simulink library "inp"  (R2024a)
settings: Solver=VariableStepAuto  StartTime=0.0  StopTime=10.0  RelTol=1e-3
undefined symbols (not defined in the file): C_TASK_5MS_S, TRUE
libraries: FVT_lib x54, hcu_lib x1
(part 1 of 2)
settings Model: Creator=13168  LastModifiedBy=FVT22063
settings SolverCC: AlgebraicLoopSolver=TrustRegion
settings DataIOCC: SaveFormat=Array  SignalLoggingSaveFormat=ModelDataLogs  ReturnWorkspaceOutputs=off
settings OptimizationCC: BlockReduction=off  BooleanDataType=off
settings DebuggingCC: SaveWithParameterizedLinksMsg=none  UnderspecifiedInitializationDetection=Classic  MergeDetectMultiDrivingBlocksExec=none  SignalResolutionControl=TryResolveAllWithWarning  UnconnectedInputMsg=warning  UnconnectedOutputMsg=warning  UnconnectedLineMsg=warning
settings HardwareCC: TargetUnknown=on
settings ModelReferenceCC: EnableRefExpFcnMdlSchedulingChecks=on  PropagateSignalLabelsOutOfModel=off
settings SFSimCC: SimUseLocalCustomCode=off
settings RTWCC: GPUComputeCapability=3.5  DLArmComputeVersion=19.05
settings ConfigComp: CovMetricSettings=dw  CovSaveCumulativeToWorkspaceVar=on  CovSaveSingleToWorkspaceVar=on

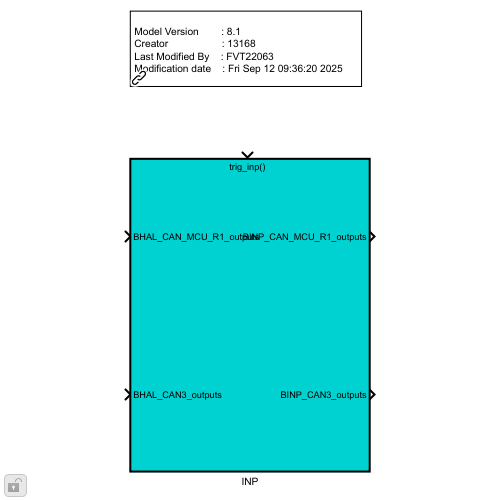
[thumbnail: Simulink's stored preview of the top-level diagram]
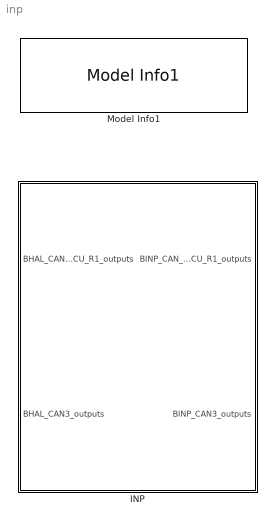
== system inp ==
  INP : Subsystem  TreatAsAtomicUnit=on
      settings: RTWSystemCode=Nonreusable function  RTWFcnNameOpts=Use subsystem name  RTWFileNameOpts=Use subsystem name
  Model Info1 : hcu_lib/Model Info1  BlockCM=None  Frame=on  DisplayStringWithTags=|  HorizontalTextAlignment=Left  LeftAlignmentValue=0.02  SourceBlockDiagram=hcu_lib  TagMaxNumber=20
      | Model Version        : %<ModelVersion>
      | Creator                   : %<Creator>
      | Last Modified By    : %<LastModifiedBy>
      | Modification date    : %<LastModificationDate>
      settings: SourceProductName=HCU Relative Block Library

== system inp/INP ==
  BHAL_CAN_MCU_R1_outputs : Inport  OutDataTypeStr=Bus: BHAL_CAN_MCU_R1_outputs
  BHAL_CAN3_outputs : Inport  Port=2  OutDataTypeStr=Bus: BHAL_CAN3_outputs
  CAN3 : Subsystem
  CAN_MCU_R1 : Subsystem
  BINP_CAN_MCU_R1_outputs : Outport  OutDataTypeStr=Bus: BINP_CAN_MCU_R1_outputs
  BINP_CAN3_outputs : Outport  Port=2  OutDataTypeStr=Bus: BINP_CAN3_outputs
  wires:
  BHAL_CAN_MCU_R1_outputs/1 -> CAN_MCU_R1/1(BHAL_CAN_MCU_R1_outputs)
  CAN_MCU_R1/1(INP_CAN_MCU_R1_outputs) -> BINP_CAN_MCU_R1_outputs/1
  BHAL_CAN3_outputs/1 -> CAN3/1(BHAL_CAN3_outputs)
  CAN3/1(INP_CAN3_outputs) -> BINP_CAN3_outputs/1

== system inp/INP/CAN3 ==
  BHAL_CAN3_outputs : Inport
  CommunicationCheck : Subsystem
  CreateBus : Subsystem
  SignalCheck : Subsystem
  ctasktime : Constant  Value=C_TASK_5MS_S  OutDataTypeStr=single
  INP_CAN3_outputs : Outport
  wires:
  CreateBus/1(BINP_outputs) -> INP_CAN3_outputs/1
  CommunicationCheck/1(inp_CanValid_bus) -> [inp_CanValid_bus], SignalCheck/1(inp_CanValid_bus)
  [inp_CanValid_bus] -> CreateBus/1(inp_CanValid_bus)
  BHAL_CAN3_outputs/1 -> CommunicationCheck/1(BHAL_outputs), SignalCheck/3(BHAL_outputs)
  SignalCheck/1(inp_Hal_bus) -> CreateBus/2(inp_Hal_bus)
  ctasktime/1 -> SignalCheck/2(TASK_TIME_S)

== system inp/INP/CAN_MCU_R1 ==
  BHAL_CAN_MCU_R1_outputs : Inport
  CommunicationCheck : Subsystem
  CreateBus : Subsystem
  SignalCheck : Subsystem
  ctasktime : Constant  Value=C_TASK_5MS_S  OutDataTypeStr=single
  INP_CAN_MCU_R1_outputs : Outport
  wires:
  CreateBus/1(BINP_outputs) -> INP_CAN_MCU_R1_outputs/1
  CommunicationCheck/1(inp_CanValid_bus) -> [inp_CanValid_bus], SignalCheck/1(inp_CanValid_bus)
  [inp_CanValid_bus] -> CreateBus/1(inp_CanValid_bus)
  BHAL_CAN_MCU_R1_outputs/1 -> CommunicationCheck/1(BHAL_outputs), SignalCheck/3(BHAL_outputs)
  SignalCheck/1(inp_Hal_bus) -> CreateBus/2(inp_Hal_bus)
  ctasktime/1 -> SignalCheck/2(TASK_TIME_S)

== system inp/INP/CAN3/CommunicationCheck ==
  BHAL_outputs : Inport
  CANMsgInvalidBMS1 : FVT_lib/inp/CAN_Msg_Validity_Process_template  SystemSampleTime=-1  VariantActivationTime=update diagram  AllowFlexibleInterface=on  Latency=0  AutoFrameSizeCalculation=off
      link override ovrdflg: Value=KINP_CANMsgInvalidBMS1_flg_ovrdflg
      link override ovrdval: Value=KINP_CANMsgInvalidBMS1_flg_ovrdval
  CANMsgInvalidBMS6 : FVT_lib/inp/CAN_Msg_Validity_Process_template  SystemSampleTime=-1  VariantActivationTime=update diagram  AllowFlexibleInterface=on  Latency=0  AutoFrameSizeCalculation=off
      link override ovrdflg: Value=KINP_CANMsgInvalidBMS6_flg_ovrdflg
      link override ovrdval: Value=KINP_CANMsgInvalidBMS6_flg_ovrdval
  CANMsgInvalidFD3C1000 : FVT_lib/inp/CAN_Msg_Validity_Process_template  SystemSampleTime=-1  VariantActivationTime=update diagram  AllowFlexibleInterface=on  Latency=0  AutoFrameSizeCalculation=off
      link override ovrdflg: Value=KINP_CANMsgInvalidFD3C1000_flg_ovrdflg
      link override ovrdval: Value=KINP_CANMsgInvalidFD3C1000_flg_ovrdval
  CANMsgInvalidFD3VCU1 : FVT_lib/inp/CAN_Msg_Validity_Process_template  SystemSampleTime=-1  VariantActivationTime=update diagram  AllowFlexibleInterface=on  Latency=0  AutoFrameSizeCalculation=off
      link override ovrdflg: Value=KINP_CANMsgInvalidFD3VCU1_flg_ovrdflg
      link override ovrdval: Value=KINP_CANMsgInvalidFD3VCU1_flg_ovrdval
  CANMsgInvalidFD3VCU2 : FVT_lib/inp/CAN_Msg_Validity_Process_template  SystemSampleTime=-1  VariantActivationTime=update diagram  AllowFlexibleInterface=on  Latency=0  AutoFrameSizeCalculation=off
      link override ovrdflg: Value=KINP_CANMsgInvalidFD3VCU2_flg_ovrdflg
      link override ovrdval: Value=KINP_CANMsgInvalidFD3VCU2_flg_ovrdval
  CANMsgInvalidFD3VCU5 : FVT_lib/inp/CAN_Msg_Validity_Process_template  SystemSampleTime=-1  VariantActivationTime=update diagram  AllowFlexibleInterface=on  Latency=0  AutoFrameSizeCalculation=off
      link override ovrdflg: Value=KINP_CANMsgInvalidFD3VCU5_flg_ovrdflg
      link override ovrdval: Value=KINP_CANMsgInvalidFD3VCU5_flg_ovrdval
  CANMsgInvalidGW3CE1000 : FVT_lib/inp/CAN_Msg_Validity_Process_template  SystemSampleTime=-1  VariantActivationTime=update diagram  AllowFlexibleInterface=on  Latency=0  AutoFrameSizeCalculation=off
      link override ovrdflg: Value=KINP_CANMsgInvalidGW3CE1000_flg_ovrdflg
      link override ovrdval: Value=KINP_CANMsgInvalidGW3CE1000_flg_ovrdval
  bus_creator : BusCreator  Inputs=7
  bus_selector : BusSelector  OutputSignals=VHAL_CANMsgInvalidBMS1_flg,VHAL_CANMsgInvalidBMS6_flg,VHAL_CANMsgInvalidFD3C1000_flg,VHAL_CANMsgInvalidFD3VCU1_flg,VHAL_CANMsgInvalidFD3VCU2_flg,VHAL_CANMsgInvalidFD3VCU5_flg,VHAL_CANMsgInvalidGW3CE1000_flg
  not{1..7} (7 alike) : Logic  Operator=NOT  AllPortsSameDT=off  OutDataTypeStr=boolean
  inp_CanValid_bus : Outport
  wires:
  BHAL_outputs/1 -> [BHAL_outputs]
  bus_selector/1 -> CANMsgInvalidBMS1/1  "<VHAL_CANMsgInvalidBMS1_flg>"
  CANMsgInvalidBMS1/1 -> not1/1
  not1/1 -> bus_creator/1  "VINP_CANMsgValidBMS1_flg"
  bus_selector/2 -> CANMsgInvalidBMS6/1  "<VHAL_CANMsgInvalidBMS6_flg>"
  CANMsgInvalidBMS6/1 -> not2/1
  not2/1 -> bus_creator/2  "VINP_CANMsgValidBMS6_flg"
  bus_selector/3 -> CANMsgInvalidFD3C1000/1  "<VHAL_CANMsgInvalidFD3C1000_flg>"
  CANMsgInvalidFD3C1000/1 -> not3/1
  not3/1 -> bus_creator/3  "VINP_CANMsgValidFD3C1000_flg"
  bus_selector/4 -> CANMsgInvalidFD3VCU1/1  "<VHAL_CANMsgInvalidFD3VCU1_flg>"
  CANMsgInvalidFD3VCU1/1 -> not4/1
  not4/1 -> bus_creator/4  "VINP_CANMsgValidFD3VCU1_flg"
  bus_selector/5 -> CANMsgInvalidFD3VCU2/1  "<VHAL_CANMsgInvalidFD3VCU2_flg>"
  CANMsgInvalidFD3VCU2/1 -> not5/1
  not5/1 -> bus_creator/5  "VINP_CANMsgValidFD3VCU2_flg"
  bus_selector/6 -> CANMsgInvalidFD3VCU5/1  "<VHAL_CANMsgInvalidFD3VCU5_flg>"
  CANMsgInvalidFD3VCU5/1 -> not6/1
  not6/1 -> bus_creator/6  "VINP_CANMsgValidFD3VCU5_flg"
  bus_selector/7 -> CANMsgInvalidGW3CE1000/1  "<VHAL_CANMsgInvalidGW3CE1000_flg>"
  CANMsgInvalidGW3CE1000/1 -> not7/1
  not7/1 -> bus_creator/7  "VINP_CANMsgValidGW3CE1000_flg"
  [BHAL_outputs] -> bus_selector/1
  bus_creator/1 -> inp_CanValid_bus/1

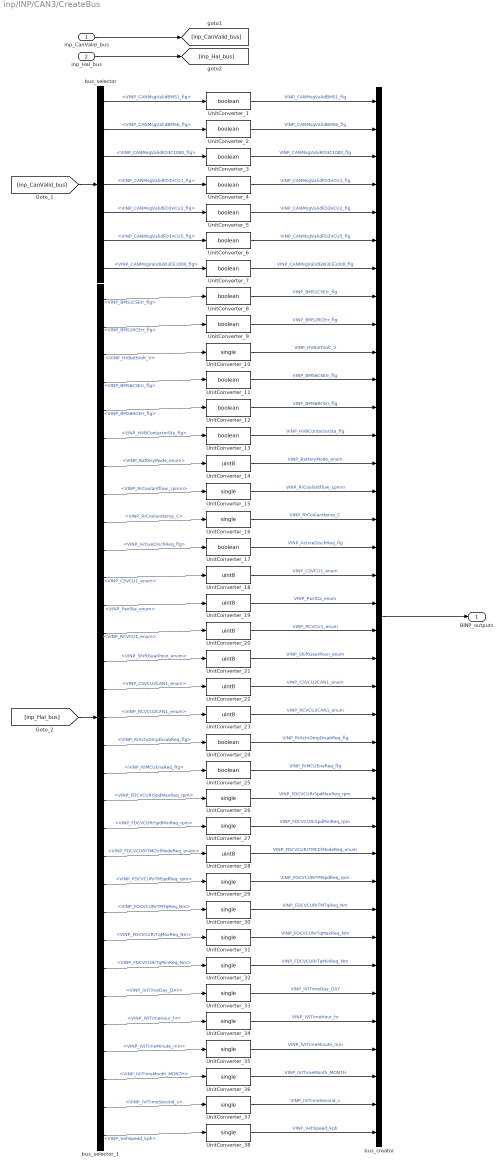
== system inp/INP/CAN3/CreateBus ==
  inp_CanValid_bus : Inport
  inp_Hal_bus : Inport  Port=2
  UnitConverter_{1..9,11..13,17,24..25} (15 alike) : DataTypeConversion  OutDataTypeStr=boolean  SaturateOnIntegerOverflow=off  RndMeth=Floor
  UnitConverter_{10,15..16,26..27,29..38} (15 alike) : DataTypeConversion  OutDataTypeStr=single  SaturateOnIntegerOverflow=off  RndMeth=Floor
  UnitConverter_{14,18..23,28} (8 alike) : DataTypeConversion  OutDataTypeStr=uint8  SaturateOnIntegerOverflow=off  RndMeth=Floor
  bus_creator : BusCreator  Inputs=38  OutDataTypeStr=Bus: BINP_CAN3_outputs  NonVirtualBus=on
  bus_selector : BusSelector  OutputSignals=VINP_CANMsgValidBMS1_flg,VINP_CANMsgValidBMS6_flg,VINP_CANMsgValidFD3C1000_flg,VINP_CANMsgValidFD3VCU1_flg,VINP_CANMsgValidFD3VCU2_flg,VINP_CANMsgValidFD3VCU5_flg,VINP_CANMsgValidGW3CE1000_flg
  bus_selector_1 : BusSelector  OutputSignals=VINP_BMS1CSErr_flg,VINP_BMS1RCErr_flg,VINP_HVBattVolt_V,VINP_BMS6CSErr_flg,VINP_BMS6RCErr_flg,VINP_HVBContactorSta_flg,VINP_BatteryMode_enum,VINP_RrCoolantflow_Lpmin,VINP_RrCoolanttemp_C,VINP_ActiveDischReq_flg,VINP_CSVCU1_enum,VINP_PwrSta_enum,VINP_RCVCU1_enum,VINP_ShiftGearPosn_enum,VINP_CSVCU2CAN1_enum,VINP_RCVCU2CAN1_enum,VINP_RrActvDmpDisabReq_flg,VINP_RrMCUEnaReq_flg,VINP_FDCVCURrSpdMaxReq_rpm,VINP_FDCVCURrSpdMinReq_rpm,VINP_FDCVCURrTMCtrlModeReq_enum,VINP_FDCVCURrTMSpdReq_rpm,VINP_FDCVCURrTMTqReq_Nm,VINP_FDCVCURrTqMaxReq_Nm,VINP_FDCVCURrTqMinReq_Nm,VINP_IVITimeDay_DAY,VINP_IVITimeHour_hr,VINP_IVITimeMinute_min,VINP_IVITimeMonth_MONTH,VINP_IVITimeSecond_s,VINP_VehSpeed_kph
  BINP_outputs : Outport
  wires:
  inp_CanValid_bus/1 -> [inp_CanValid_bus]
  inp_Hal_bus/1 -> [inp_Hal_bus]
  bus_selector/1 -> UnitConverter_1/1  "<VINP_CANMsgValidBMS1_flg>"
  UnitConverter_1/1 -> bus_creator/1  "VINP_CANMsgValidBMS1_flg"
  bus_selector/2 -> UnitConverter_2/1  "<VINP_CANMsgValidBMS6_flg>"
  UnitConverter_2/1 -> bus_creator/2  "VINP_CANMsgValidBMS6_flg"
  bus_selector/3 -> UnitConverter_3/1  "<VINP_CANMsgValidFD3C1000_flg>"
  UnitConverter_3/1 -> bus_creator/3  "VINP_CANMsgValidFD3C1000_flg"
  bus_selector/4 -> UnitConverter_4/1  "<VINP_CANMsgValidFD3VCU1_flg>"
  UnitConverter_4/1 -> bus_creator/4  "VINP_CANMsgValidFD3VCU1_flg"
  bus_selector/5 -> UnitConverter_5/1  "<VINP_CANMsgValidFD3VCU2_flg>"
  UnitConverter_5/1 -> bus_creator/5  "VINP_CANMsgValidFD3VCU2_flg"
  bus_selector/6 -> UnitConverter_6/1  "<VINP_CANMsgValidFD3VCU5_flg>"
  UnitConverter_6/1 -> bus_creator/6  "VINP_CANMsgValidFD3VCU5_flg"
  bus_selector/7 -> UnitConverter_7/1  "<VINP_CANMsgValidGW3CE1000_flg>"
  UnitConverter_7/1 -> bus_creator/7  "VINP_CANMsgValidGW3CE1000_flg"
  bus_selector_1/1 -> UnitConverter_8/1  "<VINP_BMS1CSErr_flg>"
  UnitConverter_8/1 -> bus_creator/8  "VINP_BMS1CSErr_flg"
  bus_selector_1/2 -> UnitConverter_9/1  "<VINP_BMS1RCErr_flg>"
  UnitConverter_9/1 -> bus_creator/9  "VINP_BMS1RCErr_flg"
  bus_selector_1/3 -> UnitConverter_10/1  "<VINP_HVBattVolt_V>"
  UnitConverter_10/1 -> bus_creator/10  "VINP_HVBattVolt_V"
  bus_selector_1/4 -> UnitConverter_11/1  "<VINP_BMS6CSErr_flg>"
  UnitConverter_11/1 -> bus_creator/11  "VINP_BMS6CSErr_flg"
  bus_selector_1/5 -> UnitConverter_12/1  "<VINP_BMS6RCErr_flg>"
  UnitConverter_12/1 -> bus_creator/12  "VINP_BMS6RCErr_flg"
  bus_selector_1/6 -> UnitConverter_13/1  "<VINP_HVBContactorSta_flg>"
  UnitConverter_13/1 -> bus_creator/13  "VINP_HVBContactorSta_flg"
  bus_selector_1/7 -> UnitConverter_14/1  "<VINP_BatteryMode_enum>"
  UnitConverter_14/1 -> bus_creator/14  "VINP_BatteryMode_enum"
  bus_selector_1/8 -> UnitConverter_15/1  "<VINP_RrCoolantflow_Lpmin>"
  UnitConverter_15/1 -> bus_creator/15  "VINP_RrCoolantflow_Lpmin"
  bus_selector_1/9 -> UnitConverter_16/1  "<VINP_RrCoolanttemp_C>"
  UnitConverter_16/1 -> bus_creator/16  "VINP_RrCoolanttemp_C"
  bus_selector_1/10 -> UnitConverter_17/1  "<VINP_ActiveDischReq_flg>"
  UnitConverter_17/1 -> bus_creator/17  "VINP_ActiveDischReq_flg"
  bus_selector_1/11 -> UnitConverter_18/1  "<VINP_CSVCU1_enum>"
  UnitConverter_18/1 -> bus_creator/18  "VINP_CSVCU1_enum"
  bus_selector_1/12 -> UnitConverter_19/1  "<VINP_PwrSta_enum>"
  UnitConverter_19/1 -> bus_creator/19  "VINP_PwrSta_enum"
  bus_selector_1/13 -> UnitConverter_20/1  "<VINP_RCVCU1_enum>"
  UnitConverter_20/1 -> bus_creator/20  "VINP_RCVCU1_enum"
  bus_selector_1/14 -> UnitConverter_21/1  "<VINP_ShiftGearPosn_enum>"
  UnitConverter_21/1 -> bus_creator/21  "VINP_ShiftGearPosn_enum"
  bus_selector_1/15 -> UnitConverter_22/1  "<VINP_CSVCU2CAN1_enum>"
  UnitConverter_22/1 -> bus_creator/22  "VINP_CSVCU2CAN1_enum"
  bus_selector_1/16 -> UnitConverter_23/1  "<VINP_RCVCU2CAN1_enum>"
  UnitConverter_23/1 -> bus_creator/23  "VINP_RCVCU2CAN1_enum"
  bus_selector_1/17 -> UnitConverter_24/1  "<VINP_RrActvDmpDisabReq_flg>"
  UnitConverter_24/1 -> bus_creator/24  "VINP_RrActvDmpDisabReq_flg"
  bus_selector_1/18 -> UnitConverter_25/1  "<VINP_RrMCUEnaReq_flg>"
  UnitConverter_25/1 -> bus_creator/25  "VINP_RrMCUEnaReq_flg"
  bus_selector_1/19 -> UnitConverter_26/1  "<VINP_FDCVCURrSpdMaxReq_rpm>"
  UnitConverter_26/1 -> bus_creator/26  "VINP_FDCVCURrSpdMaxReq_rpm"
  bus_selector_1/20 -> UnitConverter_27/1  "<VINP_FDCVCURrSpdMinReq_rpm>"
  UnitConverter_27/1 -> bus_creator/27  "VINP_FDCVCURrSpdMinReq_rpm"
  bus_selector_1/21 -> UnitConverter_28/1  "<VINP_FDCVCURrTMCtrlModeReq_enum>"
  UnitConverter_28/1 -> bus_creator/28  "VINP_FDCVCURrTMCtrlModeReq_enum"
  bus_selector_1/22 -> UnitConverter_29/1  "<VINP_FDCVCURrTMSpdReq_rpm>"
  UnitConverter_29/1 -> bus_creator/29  "VINP_FDCVCURrTMSpdReq_rpm"
  bus_selector_1/23 -> UnitConverter_30/1  "<VINP_FDCVCURrTMTqReq_Nm>"
  UnitConverter_30/1 -> bus_creator/30  "VINP_FDCVCURrTMTqReq_Nm"
  bus_selector_1/24 -> UnitConverter_31/1  "<VINP_FDCVCURrTqMaxReq_Nm>"
  UnitConverter_31/1 -> bus_creator/31  "VINP_FDCVCURrTqMaxReq_Nm"
  bus_selector_1/25 -> UnitConverter_32/1  "<VINP_FDCVCURrTqMinReq_Nm>"
  UnitConverter_32/1 -> bus_creator/32  "VINP_FDCVCURrTqMinReq_Nm"
  bus_selector_1/26 -> UnitConverter_33/1  "<VINP_IVITimeDay_DAY>"
  UnitConverter_33/1 -> bus_creator/33  "VINP_IVITimeDay_DAY"
  bus_selector_1/27 -> UnitConverter_34/1  "<VINP_IVITimeHour_hr>"
  UnitConverter_34/1 -> bus_creator/34  "VINP_IVITimeHour_hr"
  bus_selector_1/28 -> UnitConverter_35/1  "<VINP_IVITimeMinute_min>"
  UnitConverter_35/1 -> bus_creator/35  "VINP_IVITimeMinute_min"
  bus_selector_1/29 -> UnitConverter_36/1  "<VINP_IVITimeMonth_MONTH>"
  UnitConverter_36/1 -> bus_creator/36  "VINP_IVITimeMonth_MONTH"
  bus_selector_1/30 -> UnitConverter_37/1  "<VINP_IVITimeSecond_s>"
  UnitConverter_37/1 -> bus_creator/37  "VINP_IVITimeSecond_s"
  bus_selector_1/31 -> UnitConverter_38/1  "<VINP_VehSpeed_kph>"
  UnitConverter_38/1 -> bus_creator/38  "VINP_VehSpeed_kph"
  [inp_CanValid_bus] -> bus_selector/1
  [inp_Hal_bus] -> bus_selector_1/1
  bus_creator/1 -> BINP_outputs/1

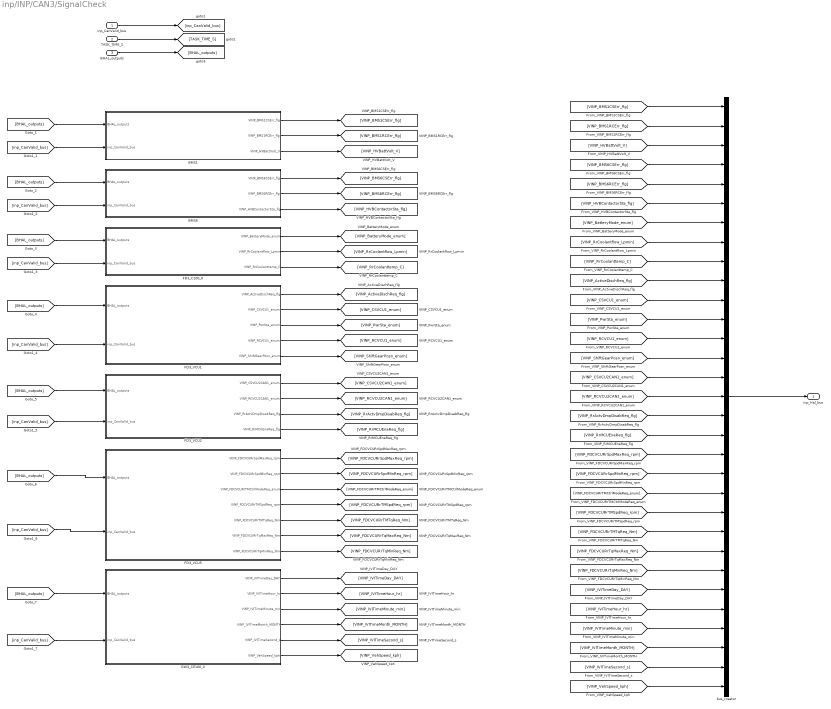
== system inp/INP/CAN3/SignalCheck ==
  inp_CanValid_bus : Inport
  TASK_TIME_S : Inport  Port=2
  BHAL_outputs : Inport  Port=3
  BMS1 : Subsystem
  BMS6 : Subsystem
  FD3_C100_0 : Subsystem
  FD3_VCU1 : Subsystem
  FD3_VCU2 : Subsystem
  FD3_VCU5 : Subsystem
  GW3_CE100_0 : Subsystem
  bus_creator : BusCreator  Inputs=31
  inp_Hal_bus : Outport
  wires:
  inp_CanValid_bus/1 -> [inp_CanValid_bus]
  TASK_TIME_S/1 -> [TASK_TIME_S]
  BHAL_outputs/1 -> [BHAL_outputs]
  [BHAL_outputs] -> BMS1/1(BHAL_outputs)
  [inp_CanValid_bus] -> BMS1/2(inp_CanValid_bus)
  BMS1/1(VINP_BMS1CSErr_flg) -> [VINP_BMS1CSErr_flg]
  BMS1/2(VINP_BMS1RCErr_flg) -> [VINP_BMS1RCErr_flg]
  BMS1/3(VINP_HVBattVolt_V) -> [VINP_HVBattVolt_V]
  [BHAL_outputs] -> BMS6/1(BHAL_outputs)
  [inp_CanValid_bus] -> BMS6/2(inp_CanValid_bus)
  BMS6/1(VINP_BMS6CSErr_flg) -> [VINP_BMS6CSErr_flg]
  BMS6/2(VINP_BMS6RCErr_flg) -> [VINP_BMS6RCErr_flg]
  BMS6/3(VINP_HVBContactorSta_flg) -> [VINP_HVBContactorSta_flg]
  [BHAL_outputs] -> FD3_C100_0/1(BHAL_outputs)
  [inp_CanValid_bus] -> FD3_C100_0/2(inp_CanValid_bus)
  FD3_C100_0/1(VINP_BatteryMode_enum) -> [VINP_BatteryMode_enum]
  FD3_C100_0/2(VINP_RrCoolantflow_Lpmin) -> [VINP_RrCoolantflow_Lpmin]
  FD3_C100_0/3(VINP_RrCoolanttemp_C) -> [VINP_RrCoolanttemp_C]
  [BHAL_outputs] -> FD3_VCU1/1(BHAL_outputs)
  [inp_CanValid_bus] -> FD3_VCU1/2(inp_CanValid_bus)
  FD3_VCU1/1(VINP_ActiveDischReq_flg) -> [VINP_ActiveDischReq_flg]
  FD3_VCU1/2(VINP_CSVCU1_enum) -> [VINP_CSVCU1_enum]
  FD3_VCU1/3(VINP_PwrSta_enum) -> [VINP_PwrSta_enum]
  FD3_VCU1/4(VINP_RCVCU1_enum) -> [VINP_RCVCU1_enum]
  FD3_VCU1/5(VINP_ShiftGearPosn_enum) -> [VINP_ShiftGearPosn_enum]
  [BHAL_outputs] -> FD3_VCU2/1(BHAL_outputs)
  [inp_CanValid_bus] -> FD3_VCU2/2(inp_CanValid_bus)
  FD3_VCU2/1(VINP_CSVCU2CAN1_enum) -> [VINP_CSVCU2CAN1_enum]
  FD3_VCU2/2(VINP_RCVCU2CAN1_enum) -> [VINP_RCVCU2CAN1_enum]
  FD3_VCU2/3(VINP_RrActvDmpDisabReq_flg) -> [VINP_RrActvDmpDisabReq_flg]
  FD3_VCU2/4(VINP_RrMCUEnaReq_flg) -> [VINP_RrMCUEnaReq_flg]
  [BHAL_outputs] -> FD3_VCU5/1(BHAL_outputs)
  [inp_CanValid_bus] -> FD3_VCU5/2(inp_CanValid_bus)
  FD3_VCU5/1(VINP_FDCVCURrSpdMaxReq_rpm) -> [VINP_FDCVCURrSpdMaxReq_rpm]
  FD3_VCU5/2(VINP_FDCVCURrSpdMinReq_rpm) -> [VINP_FDCVCURrSpdMinReq_rpm]
  FD3_VCU5/3(VINP_FDCVCURrTMCtrlModeReq_enum) -> [VINP_FDCVCURrTMCtrlModeReq_enum]
  FD3_VCU5/4(VINP_FDCVCURrTMSpdReq_rpm) -> [VINP_FDCVCURrTMSpdReq_rpm]
  FD3_VCU5/5(VINP_FDCVCURrTMTqReq_Nm) -> [VINP_FDCVCURrTMTqReq_Nm]
  FD3_VCU5/6(VINP_FDCVCURrTqMaxReq_Nm) -> [VINP_FDCVCURrTqMaxReq_Nm]
  FD3_VCU5/7(VINP_FDCVCURrTqMinReq_Nm) -> [VINP_FDCVCURrTqMinReq_Nm]
  [BHAL_outputs] -> GW3_CE100_0/1(BHAL_outputs)
  [inp_CanValid_bus] -> GW3_CE100_0/2(inp_CanValid_bus)
  GW3_CE100_0/1(VINP_IVITimeDay_DAY) -> [VINP_IVITimeDay_DAY]
  GW3_CE100_0/2(VINP_IVITimeHour_hr) -> [VINP_IVITimeHour_hr]
  GW3_CE100_0/3(VINP_IVITimeMinute_min) -> [VINP_IVITimeMinute_min]
  GW3_CE100_0/4(VINP_IVITimeMonth_MONTH) -> [VINP_IVITimeMonth_MONTH]
  GW3_CE100_0/5(VINP_IVITimeSecond_s) -> [VINP_IVITimeSecond_s]
  GW3_CE100_0/6(VINP_VehSpeed_kph) -> [VINP_VehSpeed_kph]
  bus_creator/1 -> inp_Hal_bus/1
  [VINP_BMS1CSErr_flg] -> bus_creator/1
  [VINP_BMS1RCErr_flg] -> bus_creator/2
  [VINP_HVBattVolt_V] -> bus_creator/3
  [VINP_BMS6CSErr_flg] -> bus_creator/4
  [VINP_BMS6RCErr_flg] -> bus_creator/5
  [VINP_HVBContactorSta_flg] -> bus_creator/6
  [VINP_BatteryMode_enum] -> bus_creator/7
  [VINP_RrCoolantflow_Lpmin] -> bus_creator/8
  [VINP_RrCoolanttemp_C] -> bus_creator/9
  [VINP_ActiveDischReq_flg] -> bus_creator/10
  [VINP_CSVCU1_enum] -> bus_creator/11
  [VINP_PwrSta_enum] -> bus_creator/12
  [VINP_RCVCU1_enum] -> bus_creator/13
  [VINP_ShiftGearPosn_enum] -> bus_creator/14
  [VINP_CSVCU2CAN1_enum] -> bus_creator/15
  [VINP_RCVCU2CAN1_enum] -> bus_creator/16
  [VINP_RrActvDmpDisabReq_flg] -> bus_creator/17
  [VINP_RrMCUEnaReq_flg] -> bus_creator/18
  [VINP_FDCVCURrSpdMaxReq_rpm] -> bus_creator/19
  [VINP_FDCVCURrSpdMinReq_rpm] -> bus_creator/20
  [VINP_FDCVCURrTMCtrlModeReq_enum] -> bus_creator/21
  [VINP_FDCVCURrTMSpdReq_rpm] -> bus_creator/22
  [VINP_FDCVCURrTMTqReq_Nm] -> bus_creator/23
  [VINP_FDCVCURrTqMaxReq_Nm] -> bus_creator/24
  [VINP_FDCVCURrTqMinReq_Nm] -> bus_creator/25
  [VINP_IVITimeDay_DAY] -> bus_creator/26
  [VINP_IVITimeHour_hr] -> bus_creator/27
  [VINP_IVITimeMinute_min] -> bus_creator/28
  [VINP_IVITimeMonth_MONTH] -> bus_creator/29
  [VINP_IVITimeSecond_s] -> bus_creator/30
  [VINP_VehSpeed_kph] -> bus_creator/31

== system inp/INP/CAN_MCU_R1/CommunicationCheck ==
  BHAL_outputs : Inport
  CANMsgInvalidEOPFVTRLocal1 : FVT_lib/inp/CAN_Msg_Validity_Process_template  SystemSampleTime=-1  VariantActivationTime=update diagram  AllowFlexibleInterface=on  Latency=0  AutoFrameSizeCalculation=off
      link override ovrdflg: Value=KINP_CANMsgInvalidEOPFVTRLocal1_flg_ovrdflg
      link override ovrdval: Value=KINP_CANMsgInvalidEOPFVTRLocal1_flg_ovrdval
  bus_creator : BusCreator  Inputs=1
  bus_selector : BusSelector  OutputSignals=VHAL_CANMsgInvalidEOPFVTRLocal1_flg
  not1 : Logic  Operator=NOT  AllPortsSameDT=off  OutDataTypeStr=boolean
  inp_CanValid_bus : Outport
  wires:
  BHAL_outputs/1 -> [BHAL_outputs]
  bus_selector/1 -> CANMsgInvalidEOPFVTRLocal1/1  "<VHAL_CANMsgInvalidEOPFVTRLocal1_flg>"
  CANMsgInvalidEOPFVTRLocal1/1 -> not1/1
  not1/1 -> bus_creator/1  "VINP_CANMsgValidEOPFVTRLocal1_flg"
  [BHAL_outputs] -> bus_selector/1
  bus_creator/1 -> inp_CanValid_bus/1

== system inp/INP/CAN_MCU_R1/CreateBus ==
  inp_CanValid_bus : Inport
  inp_Hal_bus : Inport  Port=2
  UnitConverter_{1,3..6,10,12..13,15} (9 alike) : DataTypeConversion  OutDataTypeStr=boolean  SaturateOnIntegerOverflow=off  RndMeth=Floor
  UnitConverter_{7..9,11,14,16} (6 alike) : DataTypeConversion  OutDataTypeStr=uint8  SaturateOnIntegerOverflow=off  RndMeth=Floor
  UnitConverter_2 : DataTypeConversion  OutDataTypeStr=single  SaturateOnIntegerOverflow=off  RndMeth=Floor
  bus_creator : BusCreator  Inputs=16  OutDataTypeStr=Bus: BINP_CAN_MCU_R1_outputs  NonVirtualBus=on
  bus_selector : BusSelector  OutputSignals=VINP_CANMsgValidEOPFVTRLocal1_flg
  bus_selector_1 : BusSelector  OutputSignals=VINP_EOPFVTRActualSpdSta_rpm,VINP_EOPFVTRCSInvalidSta_flg,VINP_EOPFVTRCanLossSta_flg,VINP_EOPFVTREnableOffSta_flg,VINP_EOPFVTRHallSigErrSta_flg,VINP_EOPFVTRLocal1CSSta_enum,VINP_EOPFVTRLocal1RCSta_enum,VINP_EOPFVTROverTempBCKSta_enum,VINP_EOPFVTROverTempSta_flg,VINP_EOPFVTROverVolSta_enum,VINP_EOPFVTRPumpReadySta_flg,VINP_EOPFVTRRCInvalidSta_flg,VINP_EOPFVTRRunStatusSta_enum,VINP_EOPFVTRStartFailureSta_flg,VINP_EOPFVTRUnderVolSta_enum
  BINP_outputs : Outport
  wires:
  inp_CanValid_bus/1 -> [inp_CanValid_bus]
  inp_Hal_bus/1 -> [inp_Hal_bus]
  bus_selector/1 -> UnitConverter_1/1  "<VINP_CANMsgValidEOPFVTRLocal1_flg>"
  UnitConverter_1/1 -> bus_creator/1  "VINP_CANMsgValidEOPFVTRLocal1_flg"
  bus_selector_1/1 -> UnitConverter_2/1  "<VINP_EOPFVTRActualSpdSta_rpm>"
  UnitConverter_2/1 -> bus_creator/2  "VINP_EOPFVTRActualSpdSta_rpm"
  bus_selector_1/2 -> UnitConverter_3/1  "<VINP_EOPFVTRCSInvalidSta_flg>"
  UnitConverter_3/1 -> bus_creator/3  "VINP_EOPFVTRCSInvalidSta_flg"
  bus_selector_1/3 -> UnitConverter_4/1  "<VINP_EOPFVTRCanLossSta_flg>"
  UnitConverter_4/1 -> bus_creator/4  "VINP_EOPFVTRCanLossSta_flg"
  bus_selector_1/4 -> UnitConverter_5/1  "<VINP_EOPFVTREnableOffSta_flg>"
  UnitConverter_5/1 -> bus_creator/5  "VINP_EOPFVTREnableOffSta_flg"
  bus_selector_1/5 -> UnitConverter_6/1  "<VINP_EOPFVTRHallSigErrSta_flg>"
  UnitConverter_6/1 -> bus_creator/6  "VINP_EOPFVTRHallSigErrSta_flg"
  bus_selector_1/6 -> UnitConverter_7/1  "<VINP_EOPFVTRLocal1CSSta_enum>"
  UnitConverter_7/1 -> bus_creator/7  "VINP_EOPFVTRLocal1CSSta_enum"
  bus_selector_1/7 -> UnitConverter_8/1  "<VINP_EOPFVTRLocal1RCSta_enum>"
  UnitConverter_8/1 -> bus_creator/8  "VINP_EOPFVTRLocal1RCSta_enum"
  bus_selector_1/8 -> UnitConverter_9/1  "<VINP_EOPFVTROverTempBCKSta_enum>"
  UnitConverter_9/1 -> bus_creator/9  "VINP_EOPFVTROverTempBCKSta_enum"
  bus_selector_1/9 -> UnitConverter_10/1  "<VINP_EOPFVTROverTempSta_flg>"
  UnitConverter_10/1 -> bus_creator/10  "VINP_EOPFVTROverTempSta_flg"
  bus_selector_1/10 -> UnitConverter_11/1  "<VINP_EOPFVTROverVolSta_enum>"
  UnitConverter_11/1 -> bus_creator/11  "VINP_EOPFVTROverVolSta_enum"
  bus_selector_1/11 -> UnitConverter_12/1  "<VINP_EOPFVTRPumpReadySta_flg>"
  UnitConverter_12/1 -> bus_creator/12  "VINP_EOPFVTRPumpReadySta_flg"
  bus_selector_1/12 -> UnitConverter_13/1  "<VINP_EOPFVTRRCInvalidSta_flg>"
  UnitConverter_13/1 -> bus_creator/13  "VINP_EOPFVTRRCInvalidSta_flg"
  bus_selector_1/13 -> UnitConverter_14/1  "<VINP_EOPFVTRRunStatusSta_enum>"
  UnitConverter_14/1 -> bus_creator/14  "VINP_EOPFVTRRunStatusSta_enum"
  bus_selector_1/14 -> UnitConverter_15/1  "<VINP_EOPFVTRStartFailureSta_flg>"
  UnitConverter_15/1 -> bus_creator/15  "VINP_EOPFVTRStartFailureSta_flg"
  bus_selector_1/15 -> UnitConverter_16/1  "<VINP_EOPFVTRUnderVolSta_enum>"
  UnitConverter_16/1 -> bus_creator/16  "VINP_EOPFVTRUnderVolSta_enum"
  [inp_CanValid_bus] -> bus_selector/1
  [inp_Hal_bus] -> bus_selector_1/1
  bus_creator/1 -> BINP_outputs/1

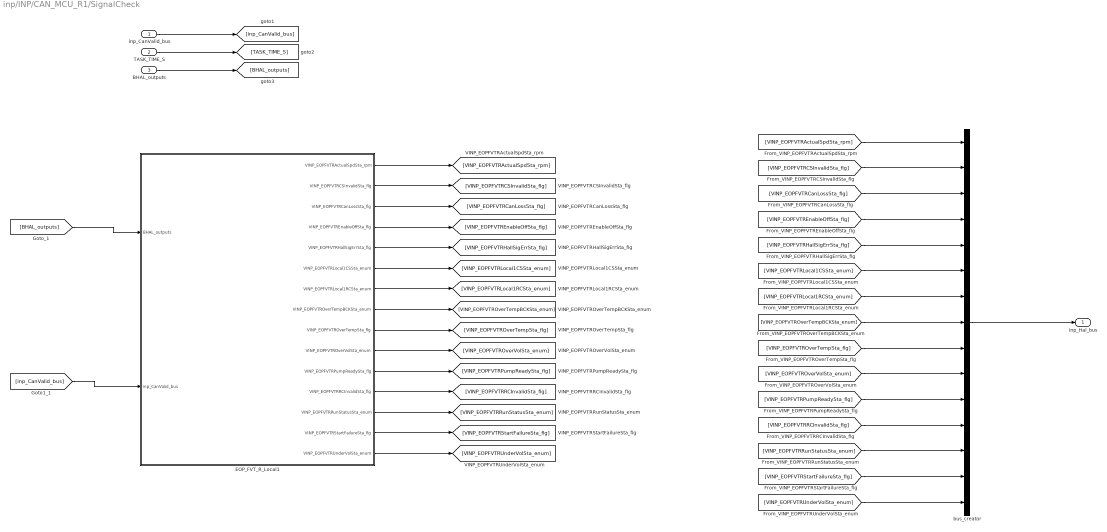
== system inp/INP/CAN_MCU_R1/SignalCheck ==
  inp_CanValid_bus : Inport
  TASK_TIME_S : Inport  Port=2
  BHAL_outputs : Inport  Port=3
  EOP_FVT_R_Local1 : Subsystem
  bus_creator : BusCreator  Inputs=15
  inp_Hal_bus : Outport
  wires:
  inp_CanValid_bus/1 -> [inp_CanValid_bus]
  TASK_TIME_S/1 -> [TASK_TIME_S]
  BHAL_outputs/1 -> [BHAL_outputs]
  [BHAL_outputs] -> EOP_FVT_R_Local1/1(BHAL_outputs)
  [inp_CanValid_bus] -> EOP_FVT_R_Local1/2(inp_CanValid_bus)
  EOP_FVT_R_Local1/1(VINP_EOPFVTRActualSpdSta_rpm) -> [VINP_EOPFVTRActualSpdSta_rpm]
  EOP_FVT_R_Local1/2(VINP_EOPFVTRCSInvalidSta_flg) -> [VINP_EOPFVTRCSInvalidSta_flg]
  EOP_FVT_R_Local1/3(VINP_EOPFVTRCanLossSta_flg) -> [VINP_EOPFVTRCanLossSta_flg]
  EOP_FVT_R_Local1/4(VINP_EOPFVTREnableOffSta_flg) -> [VINP_EOPFVTREnableOffSta_flg]
  EOP_FVT_R_Local1/5(VINP_EOPFVTRHallSigErrSta_flg) -> [VINP_EOPFVTRHallSigErrSta_flg]
  EOP_FVT_R_Local1/6(VINP_EOPFVTRLocal1CSSta_enum) -> [VINP_EOPFVTRLocal1CSSta_enum]
  EOP_FVT_R_Local1/7(VINP_EOPFVTRLocal1RCSta_enum) -> [VINP_EOPFVTRLocal1RCSta_enum]
  EOP_FVT_R_Local1/8(VINP_EOPFVTROverTempBCKSta_enum) -> [VINP_EOPFVTROverTempBCKSta_enum]
  EOP_FVT_R_Local1/9(VINP_EOPFVTROverTempSta_flg) -> [VINP_EOPFVTROverTempSta_flg]
  EOP_FVT_R_Local1/10(VINP_EOPFVTROverVolSta_enum) -> [VINP_EOPFVTROverVolSta_enum]
  EOP_FVT_R_Local1/11(VINP_EOPFVTRPumpReadySta_flg) -> [VINP_EOPFVTRPumpReadySta_flg]
  EOP_FVT_R_Local1/12(VINP_EOPFVTRRCInvalidSta_flg) -> [VINP_EOPFVTRRCInvalidSta_flg]
  EOP_FVT_R_Local1/13(VINP_EOPFVTRRunStatusSta_enum) -> [VINP_EOPFVTRRunStatusSta_enum]
  EOP_FVT_R_Local1/14(VINP_EOPFVTRStartFailureSta_flg) -> [VINP_EOPFVTRStartFailureSta_flg]
  EOP_FVT_R_Local1/15(VINP_EOPFVTRUnderVolSta_enum) -> [VINP_EOPFVTRUnderVolSta_enum]
  bus_creator/1 -> inp_Hal_bus/1
  [VINP_EOPFVTRActualSpdSta_rpm] -> bus_creator/1
  [VINP_EOPFVTRCSInvalidSta_flg] -> bus_creator/2
  [VINP_EOPFVTRCanLossSta_flg] -> bus_creator/3
  [VINP_EOPFVTREnableOffSta_flg] -> bus_creator/4
  [VINP_EOPFVTRHallSigErrSta_flg] -> bus_creator/5
  [VINP_EOPFVTRLocal1CSSta_enum] -> bus_creator/6
  [VINP_EOPFVTRLocal1RCSta_enum] -> bus_creator/7
  [VINP_EOPFVTROverTempBCKSta_enum] -> bus_creator/8
  [VINP_EOPFVTROverTempSta_flg] -> bus_creator/9
  [VINP_EOPFVTROverVolSta_enum] -> bus_creator/10
  [VINP_EOPFVTRPumpReadySta_flg] -> bus_creator/11
  [VINP_EOPFVTRRCInvalidSta_flg] -> bus_creator/12
  [VINP_EOPFVTRRunStatusSta_enum] -> bus_creator/13
  [VINP_EOPFVTRStartFailureSta_flg] -> bus_creator/14
  [VINP_EOPFVTRUnderVolSta_enum] -> bus_creator/15

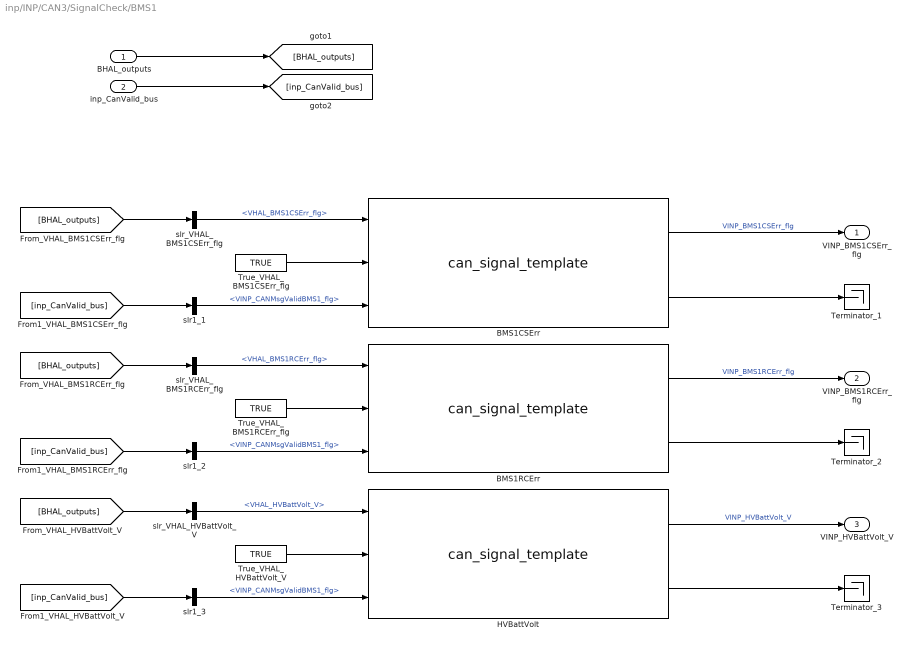
== system inp/INP/CAN3/SignalCheck/BMS1 ==
  BHAL_outputs : Inport
  inp_CanValid_bus : Inport  Port=2
  BMS1CSErr : FVT_lib/inp/can_signal_template  SystemSampleTime=-1  VariantActivationTime=update diagram  AllowFlexibleInterface=on  Latency=0  AutoFrameSizeCalculation=off
      link override defval: Value=KINP_BMS1CSErr_flg_defval
      link override ovrdflg: Value=KINP_BMS1CSErr_flg_ovrdflg
      link override ovrdval: Value=KINP_BMS1CSErr_flg_ovrdval
  BMS1RCErr : FVT_lib/inp/can_signal_template  SystemSampleTime=-1  VariantActivationTime=update diagram  AllowFlexibleInterface=on  Latency=0  AutoFrameSizeCalculation=off
      link override defval: Value=KINP_BMS1RCErr_flg_defval
      link override ovrdflg: Value=KINP_BMS1RCErr_flg_ovrdflg
      link override ovrdval: Value=KINP_BMS1RCErr_flg_ovrdval
  HVBattVolt : FVT_lib/inp/can_signal_template  SystemSampleTime=-1  VariantActivationTime=update diagram  AllowFlexibleInterface=on  Latency=0  AutoFrameSizeCalculation=off
      link override defval: Value=KINP_HVBattVolt_V_defval
      link override ovrdflg: Value=KINP_HVBattVolt_V_ovrdflg
      link override ovrdval: Value=KINP_HVBattVolt_V_ovrdval
  Terminator_1 : Terminator
  Terminator_2 : Terminator
  Terminator_3 : Terminator
  True_VHAL_BMS1CSErr_flg : Constant  Value=TRUE  OutDataTypeStr=boolean
  True_VHAL_BMS1RCErr_flg : Constant  Value=TRUE  OutDataTypeStr=boolean
  True_VHAL_HVBattVolt_V : Constant  Value=TRUE  OutDataTypeStr=boolean
  slr1_1 : BusSelector  OutputSignals=VINP_CANMsgValidBMS1_flg
  slr1_2 : BusSelector  OutputSignals=VINP_CANMsgValidBMS1_flg
  slr1_3 : BusSelector  OutputSignals=VINP_CANMsgValidBMS1_flg
  slr_VHAL_BMS1CSErr_flg : BusSelector  OutputSignals=VHAL_BMS1CSErr_flg
  slr_VHAL_BMS1RCErr_flg : BusSelector  OutputSignals=VHAL_BMS1RCErr_flg
  slr_VHAL_HVBattVolt_V : BusSelector  OutputSignals=VHAL_HVBattVolt_V
  VINP_BMS1CSErr_flg : Outport
  VINP_BMS1RCErr_flg : Outport  Port=2
  VINP_HVBattVolt_V : Outport  Port=3
  wires:
  BHAL_outputs/1 -> [BHAL_outputs]
  inp_CanValid_bus/1 -> [inp_CanValid_bus]
  [BHAL_outputs] -> slr_VHAL_BMS1CSErr_flg/1
  slr_VHAL_BMS1CSErr_flg/1 -> BMS1CSErr/1  "<VHAL_BMS1CSErr_flg>"
  True_VHAL_BMS1CSErr_flg/1 -> BMS1CSErr/2
  [inp_CanValid_bus] -> slr1_1/1
  slr1_1/1 -> BMS1CSErr/3  "<VINP_CANMsgValidBMS1_flg>"
  BMS1CSErr/1 -> VINP_BMS1CSErr_flg/1  "VINP_BMS1CSErr_flg"
  BMS1CSErr/2 -> Terminator_1/1
  [BHAL_outputs] -> slr_VHAL_BMS1RCErr_flg/1
  slr_VHAL_BMS1RCErr_flg/1 -> BMS1RCErr/1  "<VHAL_BMS1RCErr_flg>"
  True_VHAL_BMS1RCErr_flg/1 -> BMS1RCErr/2
  [inp_CanValid_bus] -> slr1_2/1
  slr1_2/1 -> BMS1RCErr/3  "<VINP_CANMsgValidBMS1_flg>"
  BMS1RCErr/1 -> VINP_BMS1RCErr_flg/1  "VINP_BMS1RCErr_flg"
  BMS1RCErr/2 -> Terminator_2/1
  [BHAL_outputs] -> slr_VHAL_HVBattVolt_V/1
  slr_VHAL_HVBattVolt_V/1 -> HVBattVolt/1  "<VHAL_HVBattVolt_V>"
  True_VHAL_HVBattVolt_V/1 -> HVBattVolt/2
  [inp_CanValid_bus] -> slr1_3/1
  slr1_3/1 -> HVBattVolt/3  "<VINP_CANMsgValidBMS1_flg>"
  HVBattVolt/1 -> VINP_HVBattVolt_V/1  "VINP_HVBattVolt_V"
  HVBattVolt/2 -> Terminator_3/1

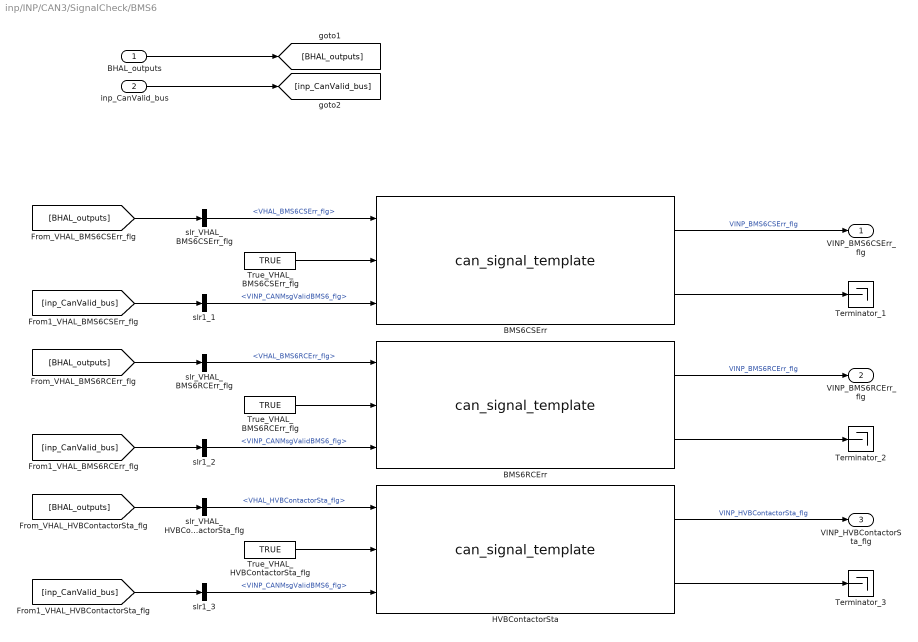
== system inp/INP/CAN3/SignalCheck/BMS6 ==
  BHAL_outputs : Inport
  inp_CanValid_bus : Inport  Port=2
  BMS6CSErr : FVT_lib/inp/can_signal_template  SystemSampleTime=-1  VariantActivationTime=update diagram  AllowFlexibleInterface=on  Latency=0  AutoFrameSizeCalculation=off
      link override defval: Value=KINP_BMS6CSErr_flg_defval
      link override ovrdflg: Value=KINP_BMS6CSErr_flg_ovrdflg
      link override ovrdval: Value=KINP_BMS6CSErr_flg_ovrdval
  BMS6RCErr : FVT_lib/inp/can_signal_template  SystemSampleTime=-1  VariantActivationTime=update diagram  AllowFlexibleInterface=on  Latency=0  AutoFrameSizeCalculation=off
      link override defval: Value=KINP_BMS6RCErr_flg_defval
      link override ovrdflg: Value=KINP_BMS6RCErr_flg_ovrdflg
      link override ovrdval: Value=KINP_BMS6RCErr_flg_ovrdval
  HVBContactorSta : FVT_lib/inp/can_signal_template  SystemSampleTime=-1  VariantActivationTime=update diagram  AllowFlexibleInterface=on  Latency=0  AutoFrameSizeCalculation=off
      link override defval: Value=KINP_HVBContactorSta_flg_defval
      link override ovrdflg: Value=KINP_HVBContactorSta_flg_ovrdflg
      link override ovrdval: Value=KINP_HVBContactorSta_flg_ovrdval
  Terminator_1 : Terminator
  Terminator_2 : Terminator
  Terminator_3 : Terminator
  True_VHAL_BMS6CSErr_flg : Constant  Value=TRUE  OutDataTypeStr=boolean
  True_VHAL_BMS6RCErr_flg : Constant  Value=TRUE  OutDataTypeStr=boolean
  True_VHAL_HVBContactorSta_flg : Constant  Value=TRUE  OutDataTypeStr=boolean
  slr1_1 : BusSelector  OutputSignals=VINP_CANMsgValidBMS6_flg
  slr1_2 : BusSelector  OutputSignals=VINP_CANMsgValidBMS6_flg
  slr1_3 : BusSelector  OutputSignals=VINP_CANMsgValidBMS6_flg
  slr_VHAL_BMS6CSErr_flg : BusSelector  OutputSignals=VHAL_BMS6CSErr_flg
  slr_VHAL_BMS6RCErr_flg : BusSelector  OutputSignals=VHAL_BMS6RCErr_flg
  slr_VHAL_HVBContactorSta_flg : BusSelector  OutputSignals=VHAL_HVBContactorSta_flg
  VINP_BMS6CSErr_flg : Outport
  VINP_BMS6RCErr_flg : Outport  Port=2
  VINP_HVBContactorSta_flg : Outport  Port=3
  wires:
  BHAL_outputs/1 -> [BHAL_outputs]
  inp_CanValid_bus/1 -> [inp_CanValid_bus]
  [BHAL_outputs] -> slr_VHAL_BMS6CSErr_flg/1
  slr_VHAL_BMS6CSErr_flg/1 -> BMS6CSErr/1  "<VHAL_BMS6CSErr_flg>"
  True_VHAL_BMS6CSErr_flg/1 -> BMS6CSErr/2
  [inp_CanValid_bus] -> slr1_1/1
  slr1_1/1 -> BMS6CSErr/3  "<VINP_CANMsgValidBMS6_flg>"
  BMS6CSErr/1 -> VINP_BMS6CSErr_flg/1  "VINP_BMS6CSErr_flg"
  BMS6CSErr/2 -> Terminator_1/1
  [BHAL_outputs] -> slr_VHAL_BMS6RCErr_flg/1
  slr_VHAL_BMS6RCErr_flg/1 -> BMS6RCErr/1  "<VHAL_BMS6RCErr_flg>"
  True_VHAL_BMS6RCErr_flg/1 -> BMS6RCErr/2
  [inp_CanValid_bus] -> slr1_2/1
  slr1_2/1 -> BMS6RCErr/3  "<VINP_CANMsgValidBMS6_flg>"
  BMS6RCErr/1 -> VINP_BMS6RCErr_flg/1  "VINP_BMS6RCErr_flg"
  BMS6RCErr/2 -> Terminator_2/1
  [BHAL_outputs] -> slr_VHAL_HVBContactorSta_flg/1
  slr_VHAL_HVBContactorSta_flg/1 -> HVBContactorSta/1  "<VHAL_HVBContactorSta_flg>"
  True_VHAL_HVBContactorSta_flg/1 -> HVBContactorSta/2
  [inp_CanValid_bus] -> slr1_3/1
  slr1_3/1 -> HVBContactorSta/3  "<VINP_CANMsgValidBMS6_flg>"
  HVBContactorSta/1 -> VINP_HVBContactorSta_flg/1  "VINP_HVBContactorSta_flg"
  HVBContactorSta/2 -> Terminator_3/1

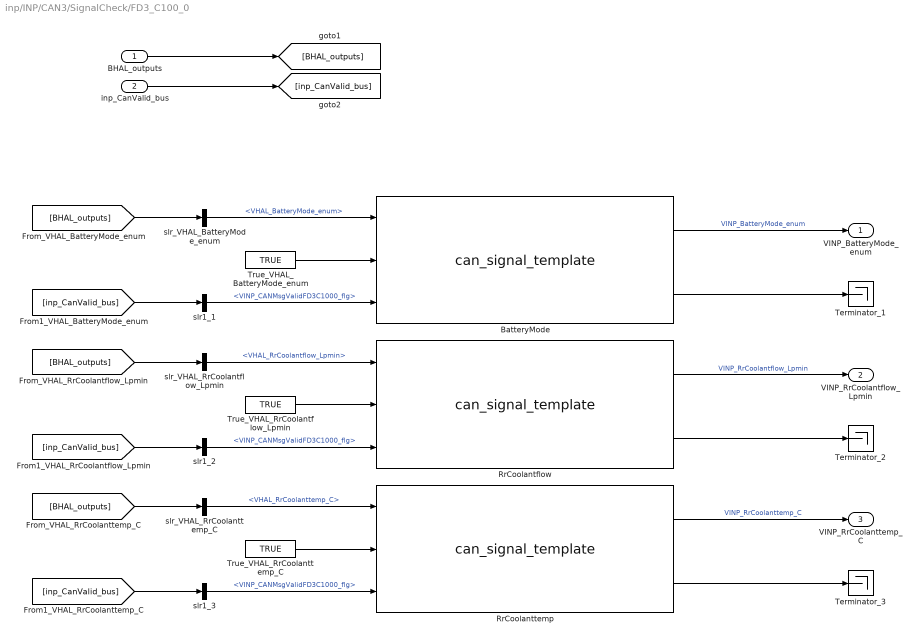
== system inp/INP/CAN3/SignalCheck/FD3_C100_0 ==
  BHAL_outputs : Inport
  inp_CanValid_bus : Inport  Port=2
  BatteryMode : FVT_lib/inp/can_signal_template  SystemSampleTime=-1  VariantActivationTime=update diagram  AllowFlexibleInterface=on  Latency=0  AutoFrameSizeCalculation=off
      link override defval: Value=KINP_BatteryMode_enum_defval
      link override ovrdflg: Value=KINP_BatteryMode_enum_ovrdflg
      link override ovrdval: Value=KINP_BatteryMode_enum_ovrdval
  RrCoolantflow : FVT_lib/inp/can_signal_template  SystemSampleTime=-1  VariantActivationTime=update diagram  AllowFlexibleInterface=on  Latency=0  AutoFrameSizeCalculation=off
      link override defval: Value=KINP_RrCoolantflow_Lpmin_defval
      link override ovrdflg: Value=KINP_RrCoolantflow_Lpmin_ovrdflg
      link override ovrdval: Value=KINP_RrCoolantflow_Lpmin_ovrdval
  RrCoolanttemp : FVT_lib/inp/can_signal_template  SystemSampleTime=-1  VariantActivationTime=update diagram  AllowFlexibleInterface=on  Latency=0  AutoFrameSizeCalculation=off
      link override defval: Value=KINP_RrCoolanttemp_C_defval
      link override ovrdflg: Value=KINP_RrCoolanttemp_C_ovrdflg
      link override ovrdval: Value=KINP_RrCoolanttemp_C_ovrdval
  Terminator_1 : Terminator
  Terminator_2 : Terminator
  Terminator_3 : Terminator
  True_VHAL_BatteryMode_enum : Constant  Value=TRUE  OutDataTypeStr=boolean
  True_VHAL_RrCoolantflow_Lpmin : Constant  Value=TRUE  OutDataTypeStr=boolean
  True_VHAL_RrCoolanttemp_C : Constant  Value=TRUE  OutDataTypeStr=boolean
  slr1_1 : BusSelector  OutputSignals=VINP_CANMsgValidFD3C1000_flg
  slr1_2 : BusSelector  OutputSignals=VINP_CANMsgValidFD3C1000_flg
  slr1_3 : BusSelector  OutputSignals=VINP_CANMsgValidFD3C1000_flg
  slr_VHAL_BatteryMode_enum : BusSelector  OutputSignals=VHAL_BatteryMode_enum
  slr_VHAL_RrCoolantflow_Lpmin : BusSelector  OutputSignals=VHAL_RrCoolantflow_Lpmin
  slr_VHAL_RrCoolanttemp_C : BusSelector  OutputSignals=VHAL_RrCoolanttemp_C
  VINP_BatteryMode_enum : Outport
  VINP_RrCoolantflow_Lpmin : Outport  Port=2
  VINP_RrCoolanttemp_C : Outport  Port=3
  wires:
  BHAL_outputs/1 -> [BHAL_outputs]
  inp_CanValid_bus/1 -> [inp_CanValid_bus]
  [BHAL_outputs] -> slr_VHAL_BatteryMode_enum/1
  slr_VHAL_BatteryMode_enum/1 -> BatteryMode/1  "<VHAL_BatteryMode_enum>"
  True_VHAL_BatteryMode_enum/1 -> BatteryMode/2
  [inp_CanValid_bus] -> slr1_1/1
  slr1_1/1 -> BatteryMode/3  "<VINP_CANMsgValidFD3C1000_flg>"
  BatteryMode/1 -> VINP_BatteryMode_enum/1  "VINP_BatteryMode_enum"
  BatteryMode/2 -> Terminator_1/1
  [BHAL_outputs] -> slr_VHAL_RrCoolantflow_Lpmin/1
  slr_VHAL_RrCoolantflow_Lpmin/1 -> RrCoolantflow/1  "<VHAL_RrCoolantflow_Lpmin>"
  True_VHAL_RrCoolantflow_Lpmin/1 -> RrCoolantflow/2
  [inp_CanValid_bus] -> slr1_2/1
  slr1_2/1 -> RrCoolantflow/3  "<VINP_CANMsgValidFD3C1000_flg>"
  RrCoolantflow/1 -> VINP_RrCoolantflow_Lpmin/1  "VINP_RrCoolantflow_Lpmin"
  RrCoolantflow/2 -> Terminator_2/1
  [BHAL_outputs] -> slr_VHAL_RrCoolanttemp_C/1
  slr_VHAL_RrCoolanttemp_C/1 -> RrCoolanttemp/1  "<VHAL_RrCoolanttemp_C>"
  True_VHAL_RrCoolanttemp_C/1 -> RrCoolanttemp/2
  [inp_CanValid_bus] -> slr1_3/1
  slr1_3/1 -> RrCoolanttemp/3  "<VINP_CANMsgValidFD3C1000_flg>"
  RrCoolanttemp/1 -> VINP_RrCoolanttemp_C/1  "VINP_RrCoolanttemp_C"
  RrCoolanttemp/2 -> Terminator_3/1

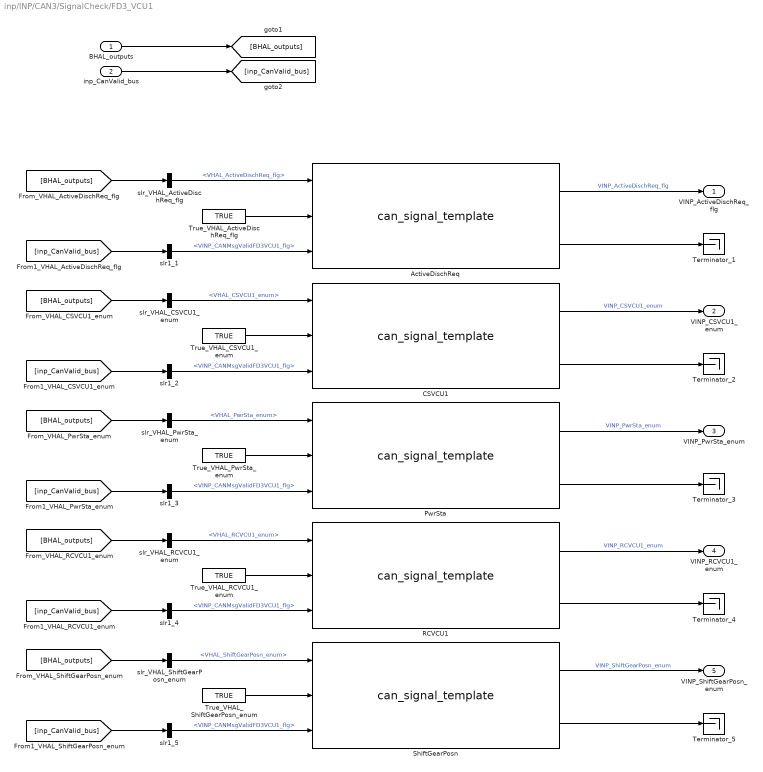
== system inp/INP/CAN3/SignalCheck/FD3_VCU1 ==
  BHAL_outputs : Inport
  inp_CanValid_bus : Inport  Port=2
  ActiveDischReq : FVT_lib/inp/can_signal_template  SystemSampleTime=-1  VariantActivationTime=update diagram  AllowFlexibleInterface=on  Latency=0  AutoFrameSizeCalculation=off
      link override defval: Value=KINP_ActiveDischReq_flg_defval
      link override ovrdflg: Value=KINP_ActiveDischReq_flg_ovrdflg
      link override ovrdval: Value=KINP_ActiveDischReq_flg_ovrdval
  CSVCU1 : FVT_lib/inp/can_signal_template  SystemSampleTime=-1  VariantActivationTime=update diagram  AllowFlexibleInterface=on  Latency=0  AutoFrameSizeCalculation=off
      link override defval: Value=KINP_CSVCU1_enum_defval
      link override ovrdflg: Value=KINP_CSVCU1_enum_ovrdflg
      link override ovrdval: Value=KINP_CSVCU1_enum_ovrdval
  PwrSta : FVT_lib/inp/can_signal_template  SystemSampleTime=-1  VariantActivationTime=update diagram  AllowFlexibleInterface=on  Latency=0  AutoFrameSizeCalculation=off
      link override defval: Value=KINP_PwrSta_enum_defval
      link override ovrdflg: Value=KINP_PwrSta_enum_ovrdflg
      link override ovrdval: Value=KINP_PwrSta_enum_ovrdval
  RCVCU1 : FVT_lib/inp/can_signal_template  SystemSampleTime=-1  VariantActivationTime=update diagram  AllowFlexibleInterface=on  Latency=0  AutoFrameSizeCalculation=off
      link override defval: Value=KINP_RCVCU1_enum_defval
      link override ovrdflg: Value=KINP_RCVCU1_enum_ovrdflg
      link override ovrdval: Value=KINP_RCVCU1_enum_ovrdval
  ShiftGearPosn : FVT_lib/inp/can_signal_template  SystemSampleTime=-1  VariantActivationTime=update diagram  AllowFlexibleInterface=on  Latency=0  AutoFrameSizeCalculation=off
      link override defval: Value=KINP_ShiftGearPosn_enum_defval
      link override ovrdflg: Value=KINP_ShiftGearPosn_enum_ovrdflg
      link override ovrdval: Value=KINP_ShiftGearPosn_enum_ovrdval
  Terminator_{1..5} (5 alike) : Terminator
  True_VHAL_ActiveDischReq_flg : Constant  Value=TRUE  OutDataTypeStr=boolean
  True_VHAL_CSVCU1_enum : Constant  Value=TRUE  OutDataTypeStr=boolean
  True_VHAL_PwrSta_enum : Constant  Value=TRUE  OutDataTypeStr=boolean
  True_VHAL_RCVCU1_enum : Constant  Value=TRUE  OutDataTypeStr=boolean
  True_VHAL_ShiftGearPosn_enum : Constant  Value=TRUE  OutDataTypeStr=boolean
  slr1_{1..5} (5 alike) : BusSelector  OutputSignals=VINP_CANMsgValidFD3VCU1_flg
  slr_VHAL_ActiveDischReq_flg : BusSelector  OutputSignals=VHAL_ActiveDischReq_flg
  slr_VHAL_CSVCU1_enum : BusSelector  OutputSignals=VHAL_CSVCU1_enum
  slr_VHAL_PwrSta_enum : BusSelector  OutputSignals=VHAL_PwrSta_enum
  slr_VHAL_RCVCU1_enum : BusSelector  OutputSignals=VHAL_RCVCU1_enum
  slr_VHAL_ShiftGearPosn_enum : BusSelector  OutputSignals=VHAL_ShiftGearPosn_enum
  VINP_ActiveDischReq_flg : Outport
  VINP_CSVCU1_enum : Outport  Port=2
  VINP_PwrSta_enum : Outport  Port=3
  VINP_RCVCU1_enum : Outport  Port=4
  VINP_ShiftGearPosn_enum : Outport  Port=5
  wires:
  BHAL_outputs/1 -> [BHAL_outputs]
  inp_CanValid_bus/1 -> [inp_CanValid_bus]
  [BHAL_outputs] -> slr_VHAL_ActiveDischReq_flg/1
  slr_VHAL_ActiveDischReq_flg/1 -> ActiveDischReq/1  "<VHAL_ActiveDischReq_flg>"
  True_VHAL_ActiveDischReq_flg/1 -> ActiveDischReq/2
  [inp_CanValid_bus] -> slr1_1/1
  slr1_1/1 -> ActiveDischReq/3  "<VINP_CANMsgValidFD3VCU1_flg>"
  ActiveDischReq/1 -> VINP_ActiveDischReq_flg/1  "VINP_ActiveDischReq_flg"
  ActiveDischReq/2 -> Terminator_1/1
  [BHAL_outputs] -> slr_VHAL_CSVCU1_enum/1
  slr_VHAL_CSVCU1_enum/1 -> CSVCU1/1  "<VHAL_CSVCU1_enum>"
  True_VHAL_CSVCU1_enum/1 -> CSVCU1/2
  [inp_CanValid_bus] -> slr1_2/1
  slr1_2/1 -> CSVCU1/3  "<VINP_CANMsgValidFD3VCU1_flg>"
  CSVCU1/1 -> VINP_CSVCU1_enum/1  "VINP_CSVCU1_enum"
  CSVCU1/2 -> Terminator_2/1
  [BHAL_outputs] -> slr_VHAL_PwrSta_enum/1
  slr_VHAL_PwrSta_enum/1 -> PwrSta/1  "<VHAL_PwrSta_enum>"
  True_VHAL_PwrSta_enum/1 -> PwrSta/2
  [inp_CanValid_bus] -> slr1_3/1
  slr1_3/1 -> PwrSta/3  "<VINP_CANMsgValidFD3VCU1_flg>"
  PwrSta/1 -> VINP_PwrSta_enum/1  "VINP_PwrSta_enum"
  PwrSta/2 -> Terminator_3/1
  [BHAL_outputs] -> slr_VHAL_RCVCU1_enum/1
  slr_VHAL_RCVCU1_enum/1 -> RCVCU1/1  "<VHAL_RCVCU1_enum>"
  True_VHAL_RCVCU1_enum/1 -> RCVCU1/2
  [inp_CanValid_bus] -> slr1_4/1
  slr1_4/1 -> RCVCU1/3  "<VINP_CANMsgValidFD3VCU1_flg>"
  RCVCU1/1 -> VINP_RCVCU1_enum/1  "VINP_RCVCU1_enum"
  RCVCU1/2 -> Terminator_4/1
  [BHAL_outputs] -> slr_VHAL_ShiftGearPosn_enum/1
  slr_VHAL_ShiftGearPosn_enum/1 -> ShiftGearPosn/1  "<VHAL_ShiftGearPosn_enum>"
  True_VHAL_ShiftGearPosn_enum/1 -> ShiftGearPosn/2
  [inp_CanValid_bus] -> slr1_5/1
  slr1_5/1 -> ShiftGearPosn/3  "<VINP_CANMsgValidFD3VCU1_flg>"
  ShiftGearPosn/1 -> VINP_ShiftGearPosn_enum/1  "VINP_ShiftGearPosn_enum"
  ShiftGearPosn/2 -> Terminator_5/1

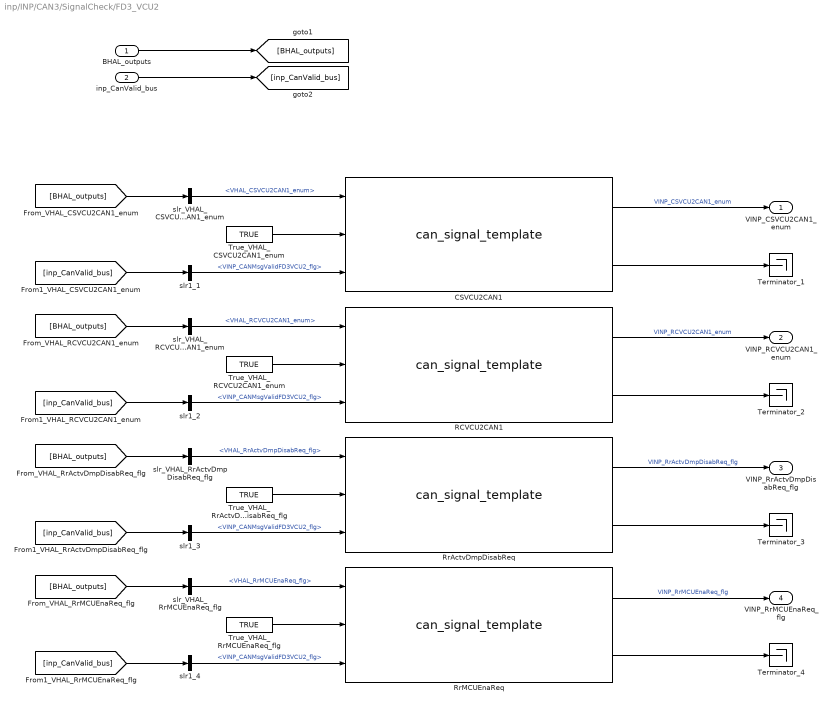
== system inp/INP/CAN3/SignalCheck/FD3_VCU2 ==
  BHAL_outputs : Inport
  inp_CanValid_bus : Inport  Port=2
  CSVCU2CAN1 : FVT_lib/inp/can_signal_template  SystemSampleTime=-1  VariantActivationTime=update diagram  AllowFlexibleInterface=on  Latency=0  AutoFrameSizeCalculation=off
      link override defval: Value=KINP_CSVCU2CAN1_enum_defval
      link override ovrdflg: Value=KINP_CSVCU2CAN1_enum_ovrdflg
      link override ovrdval: Value=KINP_CSVCU2CAN1_enum_ovrdval
  RCVCU2CAN1 : FVT_lib/inp/can_signal_template  SystemSampleTime=-1  VariantActivationTime=update diagram  AllowFlexibleInterface=on  Latency=0  AutoFrameSizeCalculation=off
      link override defval: Value=KINP_RCVCU2CAN1_enum_defval
      link override ovrdflg: Value=KINP_RCVCU2CAN1_enum_ovrdflg
      link override ovrdval: Value=KINP_RCVCU2CAN1_enum_ovrdval
  RrActvDmpDisabReq : FVT_lib/inp/can_signal_template  SystemSampleTime=-1  VariantActivationTime=update diagram  AllowFlexibleInterface=on  Latency=0  AutoFrameSizeCalculation=off
      link override defval: Value=KINP_RrActvDmpDisabReq_flg_defval
      link override ovrdflg: Value=KINP_RrActvDmpDisabReq_flg_ovrdflg
      link override ovrdval: Value=KINP_RrActvDmpDisabReq_flg_ovrdval
  RrMCUEnaReq : FVT_lib/inp/can_signal_template  SystemSampleTime=-1  VariantActivationTime=update diagram  AllowFlexibleInterface=on  Latency=0  AutoFrameSizeCalculation=off
      link override defval: Value=KINP_RrMCUEnaReq_flg_defval
      link override ovrdflg: Value=KINP_RrMCUEnaReq_flg_ovrdflg
      link override ovrdval: Value=KINP_RrMCUEnaReq_flg_ovrdval
  Terminator_{1..4} (4 alike) : Terminator
  True_VHAL_CSVCU2CAN1_enum : Constant  Value=TRUE  OutDataTypeStr=boolean
  True_VHAL_RCVCU2CAN1_enum : Constant  Value=TRUE  OutDataTypeStr=boolean
  True_VHAL_RrActvDmpDisabReq_flg : Constant  Value=TRUE  OutDataTypeStr=boolean
  True_VHAL_RrMCUEnaReq_flg : Constant  Value=TRUE  OutDataTypeStr=boolean
  slr1_{1..4} (4 alike) : BusSelector  OutputSignals=VINP_CANMsgValidFD3VCU2_flg
  slr_VHAL_CSVCU2CAN1_enum : BusSelector  OutputSignals=VHAL_CSVCU2CAN1_enum
  slr_VHAL_RCVCU2CAN1_enum : BusSelector  OutputSignals=VHAL_RCVCU2CAN1_enum
  slr_VHAL_RrActvDmpDisabReq_flg : BusSelector  OutputSignals=VHAL_RrActvDmpDisabReq_flg
  slr_VHAL_RrMCUEnaReq_flg : BusSelector  OutputSignals=VHAL_RrMCUEnaReq_flg
  VINP_CSVCU2CAN1_enum : Outport
  VINP_RCVCU2CAN1_enum : Outport  Port=2
  VINP_RrActvDmpDisabReq_flg : Outport  Port=3
  VINP_RrMCUEnaReq_flg : Outport  Port=4
  wires:
  BHAL_outputs/1 -> [BHAL_outputs]
  inp_CanValid_bus/1 -> [inp_CanValid_bus]
  [BHAL_outputs] -> slr_VHAL_CSVCU2CAN1_enum/1
  slr_VHAL_CSVCU2CAN1_enum/1 -> CSVCU2CAN1/1  "<VHAL_CSVCU2CAN1_enum>"
  True_VHAL_CSVCU2CAN1_enum/1 -> CSVCU2CAN1/2
  [inp_CanValid_bus] -> slr1_1/1
  slr1_1/1 -> CSVCU2CAN1/3  "<VINP_CANMsgValidFD3VCU2_flg>"
  CSVCU2CAN1/1 -> VINP_CSVCU2CAN1_enum/1  "VINP_CSVCU2CAN1_enum"
  CSVCU2CAN1/2 -> Terminator_1/1
  [BHAL_outputs] -> slr_VHAL_RCVCU2CAN1_enum/1
  slr_VHAL_RCVCU2CAN1_enum/1 -> RCVCU2CAN1/1  "<VHAL_RCVCU2CAN1_enum>"
  True_VHAL_RCVCU2CAN1_enum/1 -> RCVCU2CAN1/2
  [inp_CanValid_bus] -> slr1_2/1
  slr1_2/1 -> RCVCU2CAN1/3  "<VINP_CANMsgValidFD3VCU2_flg>"
  RCVCU2CAN1/1 -> VINP_RCVCU2CAN1_enum/1  "VINP_RCVCU2CAN1_enum"
  RCVCU2CAN1/2 -> Terminator_2/1
  [BHAL_outputs] -> slr_VHAL_RrActvDmpDisabReq_flg/1
  slr_VHAL_RrActvDmpDisabReq_flg/1 -> RrActvDmpDisabReq/1  "<VHAL_RrActvDmpDisabReq_flg>"
  True_VHAL_RrActvDmpDisabReq_flg/1 -> RrActvDmpDisabReq/2
  [inp_CanValid_bus] -> slr1_3/1
  slr1_3/1 -> RrActvDmpDisabReq/3  "<VINP_CANMsgValidFD3VCU2_flg>"
  RrActvDmpDisabReq/1 -> VINP_RrActvDmpDisabReq_flg/1  "VINP_RrActvDmpDisabReq_flg"
  RrActvDmpDisabReq/2 -> Terminator_3/1
  [BHAL_outputs] -> slr_VHAL_RrMCUEnaReq_flg/1
  slr_VHAL_RrMCUEnaReq_flg/1 -> RrMCUEnaReq/1  "<VHAL_RrMCUEnaReq_flg>"
  True_VHAL_RrMCUEnaReq_flg/1 -> RrMCUEnaReq/2
  [inp_CanValid_bus] -> slr1_4/1
  slr1_4/1 -> RrMCUEnaReq/3  "<VINP_CANMsgValidFD3VCU2_flg>"
  RrMCUEnaReq/1 -> VINP_RrMCUEnaReq_flg/1  "VINP_RrMCUEnaReq_flg"
  RrMCUEnaReq/2 -> Terminator_4/1
